simulink model "rHighCellTemperatureDerate"  (R2024b)
settings: configuration reference "STM32H7_Config" (kept outside this file)
settings Model: DataDictionary=Master_Dictionary.sldd  EnableAccessToBaseWorkspace=off  Creator=torni  LastModifiedBy=William
settings ConfigSetRef: SourceName=STM32H7_Config

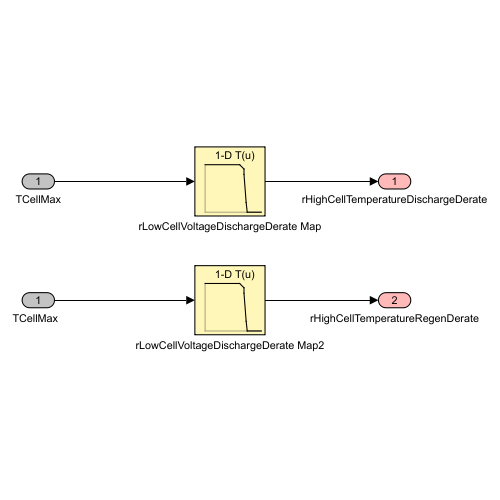
[thumbnail: Simulink's stored preview of the top-level diagram]
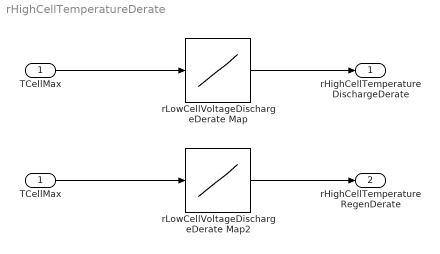
== system rHighCellTemperatureDerate ==
  "TCellMax " : Inport  OutDataTypeStr=double
  "TCellMax  " : InportShadow  OutDataTypeStr=double
  rLowCellVoltageDischargeDerate Map : Lookup_n-D  NumberOfTableDimensions=1  BreakpointsForDimension1=[0,50,55,56,58,61,80]  Table=[1,1,0.9,0.8,0.2,0,0]  InternalRulePriority=Speed  RndMeth=Simplest
  rLowCellVoltageDischargeDerate Map2 : Lookup_n-D  NumberOfTableDimensions=1  BreakpointsForDimension1=[0,50,55,56,58,61,80]  Table=[1,1,0.9,0.8,0.2,0,0]  InternalRulePriority=Speed  RndMeth=Simplest
  rHighCellTemperatureDischargeDerate : Outport  OutDataTypeStr=double  VectorParamsAs1DForOutWhenUnconnected=off
  rHighCellTemperatureRegenDerate : Outport  Port=2  OutDataTypeStr=double  VectorParamsAs1DForOutWhenUnconnected=off
  wires:
  rLowCellVoltageDischargeDerate Map/1 -> rHighCellTemperatureDischargeDerate/1
  "TCellMax "/1 -> rLowCellVoltageDischargeDerate Map/1
  rLowCellVoltageDischargeDerate Map2/1 -> rHighCellTemperatureRegenDerate/1
  "TCellMax  "/1 -> rLowCellVoltageDischargeDerate Map2/1
